simulink model "OutputCalibration_r2024a"  (R2024a)
settings: Solver=FixedStepAuto  StartTime=0.0  StopTime=inf  FixedStep=1/200  RelTol=1e-3  EnableMultiTasking=on
libraries: mbedblockslib x3
settings Model: ExtModeTrigDuration=10  Creator=patri  LastModifiedBy=Jaylen
settings SolverCC: AutoInsertRateTranBlk=on
settings OptimizationCC: EnhancedBackFolding=on  PassReuseOutputArgsAs=Individual arguments  ZeroExternalMemoryAtStartup=off  ZeroInternalMemoryAtStartup=off  MaxStackSize=64  OptimizeBlockOrder=speed  DifferentSizesBufferReuse=on  OptimizationCustomize=off  EfficientTunableParamExpr=on
settings DebuggingCC: ParameterTunabilityLossMsg=error
settings HardwareCC: ProdBitPerPointer=32  ProdBitPerSizeT=32  ProdBitPerPtrDiffT=32  ProdLargestAtomicInteger=Long  ProdLargestAtomicFloat=Double  ProdWordSize=32  ProdLongLongMode=on  ProdHWDeviceType=ARM Compatible->ARM Cortex-M
settings SFSimCC: MATLABDynamicMemAlloc=off
settings RTWCC: Description=Embedded Coder  SystemTargetFile=ert.tlc  HardwareBoard=STM32 Nucleo F767ZI  TemplateMakefile=ert_default_tmf  Toolchain=GNU Tools for ARM Embedded Processors
settings CodeAppCC: ForceParamTrailComments=on  IgnoreCustomStorageClasses=off  OperatorAnnotations=on  SimulinkDataObjDesc=on  SFDataObjDesc=on  InsertBlockDesc=on
settings ERTTargetCC: ExtModeTransport=3  ExtModeStaticAlloc=on  ExtModeStaticAllocSize=10000  ExtModeMexFile=ext_xcp  ExtModeIntrfLevel=Level2 - Open

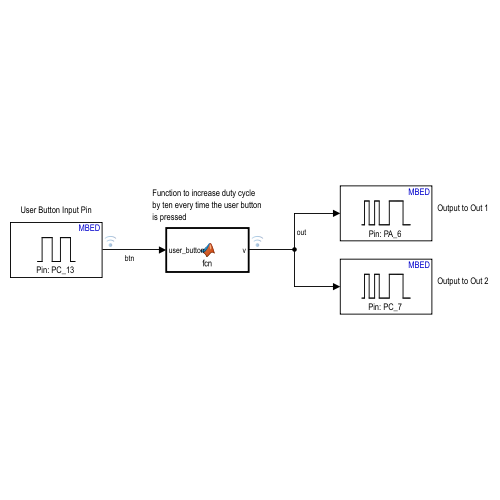
[thumbnail: Simulink's stored preview of the top-level diagram]
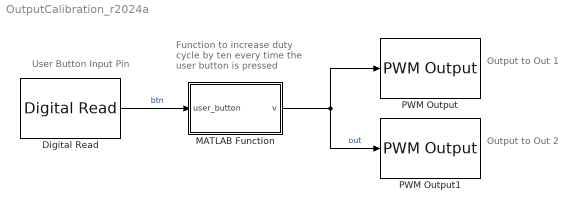
== system OutputCalibration_r2024a ==
  note: Output to Out 2
  note: Output to Out 1
  note: Function to increase duty cycle
      | by ten every time the user button
      | is pressed
  note: User Button Input Pin
  Digital Read : mbedblockslib/Digital Read  Pin=PC_13  Direction=input  SampleTime=-1
      settings: LibrarySourceBlock=stmnucleorootlib/Common/Digital Read
  MATLAB Function : MATLAB Function  TreatAsAtomicUnit=on
  PWM Output : mbedblockslib/PWM Output  Pin=PA_6  EnableInputFrequency=off  InitialFrequency=10000  InitialDutyCycle=57.6  NotificationType=None
      settings: LibrarySourceBlock=stmnucleorootlib/Common/PWM Output
  PWM Output1 : mbedblockslib/PWM Output  Pin=PC_7  EnableInputFrequency=off  InitialFrequency=10000  InitialDutyCycle=57.6  NotificationType=None
      settings: LibrarySourceBlock=stmnucleorootlib/Common/PWM Output
  wires:
  Digital Read/1 -> MATLAB Function/1(user_button)  "btn"
  MATLAB Function/1(v) -> PWM Output1/1, PWM Output/1  "out"

== matlab function OutputCalibration_r2024a/MATLAB Function ==
  data: user_button input; v output
function v = fcn(user_button)

% Create variables for the function, m is duty cycle, db if test, i is time
persistent m db i;

% Choose sample rate of 200 per second
Fs = 200;

% Set initial Values
if isempty(m)
    m = 0;
    i = 0;
    db = 0;
end

% Check if button has been pressed
if user_button == 1
    % Check if db is = 0
    if db == 0
        % Set db to 1 and add 10 to the duty cycle
        db = 1;
        m = m + 10;
    end
end

% Check if db is 1
if db == 1
    % Check if a second has passed
    if i > 1*Fs
        % Set db to 0 and reset timer
        db = 0;
        i = 0;
    else
        % Else increase timer
        i = i + 1;
    end
end

% Set output to the duty cycle
v = m;
end
